simulink model "PID_completo"  (R2022b)
settings: Solver=ode4  StartTime=0.0  StopTime=300  FixedStep=0.1  RelTol=1e-3
libraries: simulink_extras x1, realtime_pacer_lib x1
settings Model: Creator=rabai  LastModifiedBy=rabai
settings OptimizationCC: ReuseModelBlockBuffer=on

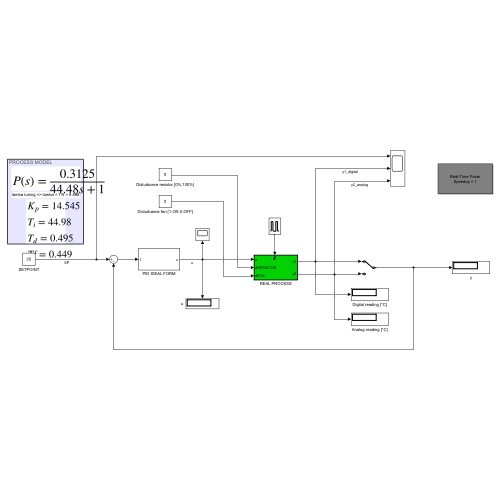
[thumbnail: Simulink's stored preview of the top-level diagram]
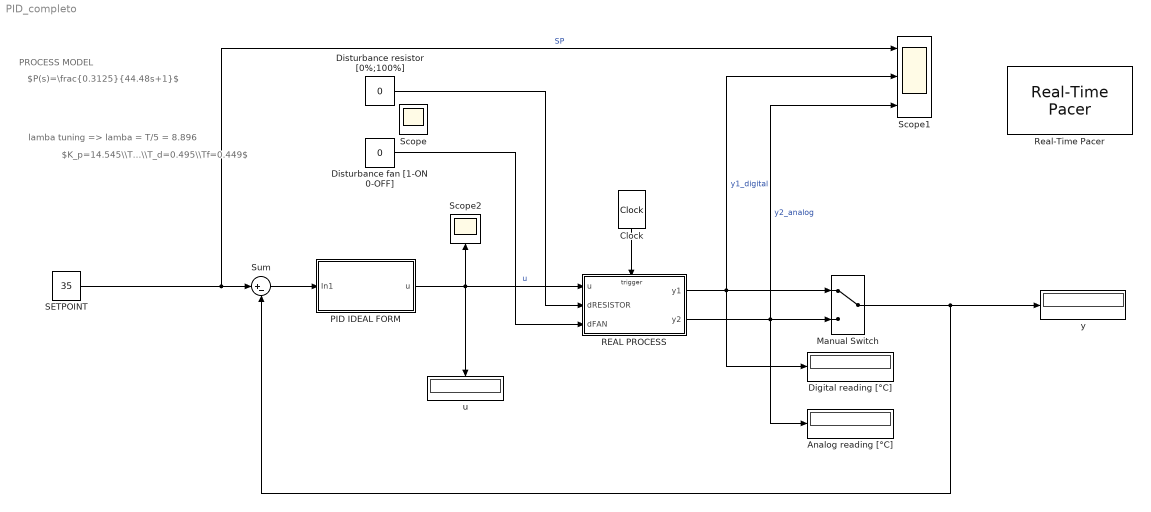
== system PID_completo ==
  note: $K_p=14.545\\T_i=44.98\\T_d=0.495\\Tf=0.449$
  note: PROCESS MODEL
  note: $P(s)=\frac{0.3125}{44.48s+1}$
  note: lamba tuning => lamba = T/5 = 8.896
  Analog reading [°C] : Display
  Clock : simulink_extras/Flip Flops/Clock  period=0.8
  Digital reading [°C] : Display
  Disturbance fan [1-ON 0-OFF] : Constant  Value=0
  Disturbance resistor [0%;100%] : Constant  Value=0
  Manual Switch : ManualSwitch
  PID IDEAL FORM : Subsystem  mask{Kp=14.59, Ti=44.98, Td=0.5, Tf=0.45}
  REAL PROCESS : Subsystem
  Real-Time Pacer : realtime_pacer_lib/Real-Time Pacer  simTimePerRealTime=1
      settings: SourceProductName=Real-Time Pacer
  SETPOINT : Constant  Value=35
  Scope1 : Scope  NumInputPorts=3
  Scope2 : Scope
  Sum : Sum  Inputs=|+-
  u : Display
  y : Display
  Scope : Scope
  wires:
  Clock/1 -> REAL PROCESS/Trigger
  Manual Switch/1 -> y/1, Sum/2
  Sum/1 -> PID IDEAL FORM/1(In1)
  PID IDEAL FORM/1(u) -> Scope2/1, REAL PROCESS/1(u), u/1  "u"
  SETPOINT/1 -> Sum/1, Scope1/1  "SP"
  Disturbance fan [1-ON 0-OFF]/1 -> REAL PROCESS/3(dFAN)
  Disturbance resistor [0%;100%]/1 -> REAL PROCESS/2(dRESISTOR)
  REAL PROCESS/1(y1) -> Digital reading [°C]/1, Scope1/2, Manual Switch/1  "y1_digital"
  REAL PROCESS/2(y2) -> Analog reading [°C]/1, Scope1/3, Manual Switch/2  "y2_analog"

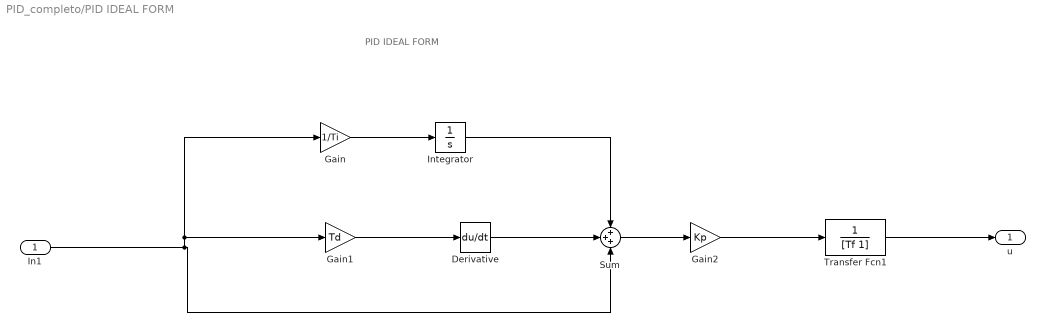
== system PID_completo/PID IDEAL FORM ==
  note: PID IDEAL FORM
  In1 : Inport
  Derivative : Derivative
  Gain : Gain  Gain=1/Ti
  Gain1 : Gain  Gain=Td
  Gain2 : Gain  Gain=Kp
  Integrator : Integrator
  Sum : Sum  Inputs=3
  Transfer Fcn1 : TransferFcn  Denominator=[Tf 1]
  u : Outport  VectorParamsAs1DForOutWhenUnconnected=off
  wires:
  Gain/1 -> Integrator/1
  Derivative/1 -> Sum/2
  Gain1/1 -> Derivative/1
  In1/1 -> Gain/1, Gain1/1, Sum/3
  Sum/1 -> Gain2/1
  Gain2/1 -> Transfer Fcn1/1
  Transfer Fcn1/1 -> u/1
  Integrator/1 -> Sum/1

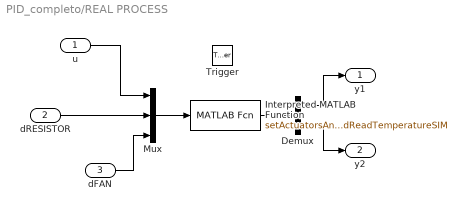
== system PID_completo/REAL PROCESS ==
  u : Inport
  dRESISTOR : Inport  Port=2
  dFAN : Inport  Port=3
  Trigger : TriggerPort  VariantControl=(inherit)  PortDimensions=1
  Demux : Demux  Outputs=2
  Interpreted MATLAB Function : MATLABFcn  MATLABFcn=setActuatorsAndReadTemperatureSIM  OutputDimensions=2
  Mux : Mux  Inputs=3
  y1 : Outport
  y2 : Outport  Port=2
  wires:
  Interpreted MATLAB Function/1 -> Demux/1
  Demux/1 -> y1/1
  Demux/2 -> y2/1
  u/1 -> Mux/1
  dRESISTOR/1 -> Mux/2
  dFAN/1 -> Mux/3
  Mux/1 -> Interpreted MATLAB Function/1
